simulink library "Lib_CanCommunication"  (R2019b)
settings: Solver=VariableStepAuto  StartTime=0.0  StopTime=10.0  RelTol=1e-3
PostLoadFcn:
  | , if any(exist('dsrtsu_mdlpostloadfcn', 'file') == [2, 3, 6]), try dsrtsu_mdlpostloadfcn('Execute', bdroot); catch fprintf('Error in PostLoadFcn (dsrtsu_mdlpostloadfcn) for model "%s":\n %s\n', bdroot, lasterr); end, end,
undefined symbols (not defined in the file): Counter, CRC, default_customer_can_bus, default_vehicle_state_bus, LateralAcceleration, LongitudinalAcceleration, Motion, Powertrain_1, Steering, steering_angle_range_rad_to_steering_wheel_angle_range_deg_gain, SteeringWheelAngle, SteeringWheelAngleSign, SteeringWheelSpeed, SteeringWheelSpeedSign, SteeringWheelTorque, SteeringWheelTorqueSign, VehicleVelocity, YawRate, YawRateSign
libraries: rtican x8, simulink x6
(part 2 of 3)

== system Lib_CanCommunication/CanCommunication/VehicleCAN/Powertrain_1Message ==
  Bus Creator : BusCreator  Inputs=8  OutDataTypeStr=Bus: Powertrain_1  NonVirtualBus=on
  Powertrain_1 : rtican/RTICAN Receive (RX)   Reserved1=[]  Reserved2=[]  Reserved3=[]  Reserved4=[]  SfcnMessage=[]  Msg_Struct=[]  BoardTypeNo=[]  BoardNo=[]  ChannelNo=[]  Parameters=[]  DialogFcn=[]  UnitName=[]  Revision=[]  UnitValues=[]  DSProperties=struct('RTI',struct('Version',uint32(5),'BlockType',struct('isSLSource',uint8(1),'isSLSink',uint8(1),'isHWSource',uint8(0),'isHWSink',uint8(0),'isSetup',uint8(0),'isInline',uint8(1),'isNonInline',uint8(0),'isInterrupt',uint8(0),'isChannelwise',uint8(0)),'IOBoardType','RTICAN','UnitType','MESSAGE','Identifier','RX','DialogType','MSVC','BlockSet','RTICAN','SlaveProcessor','CAN'))  RTIBlockInterface=struct('OutputPortsWidth',int32([1 1 1 1 1 1 1 1 1 1 1]),'OutputPortsActive',ones(1,11),'OutputPortsName',{{'CRC','Counter','Gear','ThrottlePedalPos','EngineSpeed','ActualTorqueEngine','EngineRunning','RequestedTorqueEngine',['RX status'],['RX time'],['RX delta time']}},'OutputPortsDataType',{{'SS_UINT8','SS_UINT8','SS_UINT8','SS_DOUBLE','SS_DOUBLE','SS_UINT16','SS_BOOLEAN','SS_INT16','SS_DOUBLE','SS_DOUBLE','SS_DOUBLE'}},'OutputPortsLabel',{{'CRC','Counter','Gear','ThrottlePedalPos','EngineSpeed','ActualTorqueEngine','EngineRunning','RequestedTorqueEngine','','',''}},'OutputPortsLabelMode','ON','InputPortsWidth',int32(0),'InputPortsActive',0,'DialogFcn','rtican_message_interface_gui','BlockDisplay',{{'','center'}},'IconTransparency','on','ParameterTunableNames',{{}},'InitLevel',3,'BlockName',struct('Token',{{'Powertrain_1'}}),'SampleTime',{{-1}},'TriggerPort',{{'none'}},'EnablePort',{{'none'}})  RTIBlockParameters="struct('BoardTypeNo',{{1,'OFF',[]}},'BoardNo',{{1,'ON',[1 16]}},'ChannelNo',{{2,'ON',[1 2]}},'Parameters',{{struct('DataFileSupport',struct('DataFileSelectedMaster',1,'DataFileSelectedLocal',0,'DataFileName','c:\\users\\kessler\\documents\\fav\\apollo_opensource\\modules\\dbc\\vehicledata_can_tfd7-17008-03_fortiss_gte.dbc|','DataFileDate',{{{''}}},'SelectedFile',['<no file selected>']),'Options',struct('StatusSelected',1,'TimeSelected',1,'DeltaTimeSelected',1,'BytePortSelected',0,'MessageLengthSelected',0,'TriggerPort',struct('Selected',0,'TriggerType',0),'UserCoding',struct('Selected',0,'InterfaceFile','UserDecodingFile','FcnName','UserDecodeFcn','InportSelected',0,'InportWidth',1,'OutportSelected',0,'OutportWidth',1),'EnablePortSelected',0,'SignalOnPortnameSelected',1,'UseRXService',0),'Message',struct('MsgOnBlocknameSelected',1,'MsgName','Powertrain_1','MsgIdFormat',0,'MsgId',4,'MsgLength',8,'NumSignals',8,'SampleTime',-1,'Signal',struct('SgnName',{'CRC','Counter','Gear','ThrottlePedalPos','EngineSpeed','ActualTorqueEngine','EngineRunning','RequestedTorqueEngine'},'SgnStartBit',{0,8,12,16,24,40,51,52},'SgnLength',{8,4,4,8,16,11,1,12},'SgnType',{0,0,0,0,0,0,0,0},'ModeValue',{-1,-1,-1,-1,-1,-1,-1,-1},'DataType',{0,0,0,0,0,0,0,0},'ByteLayout',{0,0,0,0,0,0,0,0},'Factor',{1,1,1,0.4,2^-2,1,1,1},'Offset',{0,0,0,0,0,0,0,-1527},'SgnComment',{{['Checksum for Powertrain_1 message:  CRC = Byte1 XOR Byte2 XOR Byte3 XOR Byte4 XOR Byte5 XOR Byte6 XOR Byte7. ']},{['Counter for Powertrain_1 message, incremented with every transmittal and periodically running from 0 to 15.']},{['Currently engaged gear. ']},{['Relative position of the throttle pedal in percent (100% = kickdown). ']},{['Engine speed in rpm. ']},{['Engine torque in Nm which is displayed in instrument cluster.']},{['Engine state.']},{['Engine torque requested by driver or ACC.']}},'SgnUnit',{'-','-','-','%','rpm','Nm','-','Nm'},'Min',{0,0,0,0,0,0,0,-1527},'Max',{255,15,15,101.6,16383,2045,1,1527},'SLDataType',{'SS_UINT8','SS_UINT8','SS_UINT8','SS_DOUBLE','SS_DOUBLE','SS_UINT16','SS_BOOLEAN','SS_INT16'}),'MsgIdNumFormat',0,'MsgComment',{{['Engine-related information.']}}),'Version',1.2,'general',struct('isFromLib',0)),'OFF',[]}},'GroupId',{{struct('Group',{{'RTICAN'}},'No',1,'Behavior',{{'NAMECHANGE'}},'BlockType',{{'SINK'}},'NameChangeFlag',0),'OFF',[]}},'SFcnRTICANMessage',{{struct('MsgType','RX','SFcnPortType','Scalar','MsgName','Powertrain_1','MsgIdFormat','STD','MsgId',4,'MsgLength',8,'NumSignals',8,'SampleTime',-1,'Signal',struct('SgnName',{'CRC','Counter','Gear','ThrottlePedalPos','EngineSpeed','ActualTorqueEngine','EngineRunning','RequestedTorqueEngine'},'SgnStartBit',{0,8,12,16,24,40,51,52},'SgnLength',{8,4,4,8,16,11,1,12},'SgnType',{'standard','standard','standard','standard','standard','standard','standard','standard'},'ModeValue',{-1,-1,-1,-1,-1,-1,-1,-1},'DataType',{['unsigned int'],['unsigned int'],['unsigned int'],['unsigned int'],['unsigned int'],['unsigned int'],['unsigned int'],['unsigned int']},'ByteLayout',{['little endian'],['little endian'],['little endian'],['little endian'],['little endian'],['little endian'],['little endian'],['little endian']},'Factor',{1,1,1,0.4,2^-2,1,1,1},'Offset',{0,0,0,0,0,0,0,-1527},'SLDataType',{'SS_UINT8','SS_UINT8','SS_UINT8','SS_DOUBLE','SS_DOUBLE','SS_UINT16','SS_BOOLEAN','SS_INT16'}),'StatusSelected','yes','TimeSelected','yes','DeltaTimeSelected','yes','BytePortSelected','no','MessageLengthSelected','no','TriggerPort',struct('Selected','no','TriggerType',0),'UserCoding',struct('Selected','no','InterfaceFile','UserDecodingFile','FcnName','UserDecodeFcn','InportSelected','no','InportWidth',1,'OutportSelected','no','OutportWidth',1),'EnablePortSelected','no','UseRXService','no','BoardType','DS1','BoardNo',1,'ControllerNo',2),'OFF',[]}},'TLCFileName',{{'rtican_rx_message','OFF',[]}})"  RTISFcnParameters=struct('SFcnRTICANMessage','struct','TLCFileName','char')  RTIBlockParaDefault=struct('BoardTypeNo',4302,'BoardNo',1,'ChannelNo',1,'Parameters',struct('DataFileSupport',struct('DataFileSelectedMaster',0,'DataFileSelectedLocal',0,'DataFileName','','DataFileDate','','SelectedFile',['<no file selected>']),'Options',struct('StatusSelected',1,'TimeSelected',1,'DeltaTimeSelected',1,'BytePortSelected',0,'MessageLengthSelected',0,'TriggerPort',struct('Selected',0,'TriggerType','rising'),'UserCoding',struct('Selected',0,'InterfaceFile','UserDecodingFile','FcnName','UserDecodeFcn','InportSelected',0,'InportWidth',1,'OutportSelected',0,'OutportWidth',1),'EnablePortSelected',0,'SignalOnPortnameSelected',1,'UseRXService',0),'Message',struct('MsgOnBlocknameSelected',0,'MsgName',['RX Message'],'MsgIdFormat',0,'MsgId',100,'MsgLength',8,'NumSignals',1,'SampleTime',-1,'Signal',struct('SgnName',['RX signal'],'SgnStartBit',0,'SgnLength',8,'SgnType',0,'ModeValue',-1,'DataType',0,'SLDataType','SS_DOUBLE','ByteLayout',0,'Factor',1,'Offset',0,'Min',0,'Max',255,'SgnComment',{{}},'SgnUnit',''),'MsgIdNumFormat',0,'MsgComment',{{''}}),'Version',1.2,'general',struct('isFromLib',1)),'GroupId',struct('Group',{{'RTICAN'}},'No',1,'Behavior',{{'NAMECHANGE'}},'BlockType',{{'SINK'}},'NameChangeFlag',0),'SFcnRTICANMessage',struct('MsgType','RX','MsgName',['RX Message'],'MsgIdFormat','STD','MsgId',100,'MsgLength',8,'NumSignals',1,'SampleTime',-1,'Signal',struct('SgnName',['RX signal'],'SgnStartBit',0,'SgnLength',8,'SgnType','standard','ModeValue',-1,'DataType',['unsigned int'],'ByteLayout',['little endian'],'SLDataType','SS_DOUBLE','Factor',1,'Offset',0),'StatusSelected','yes','TimeSelected','yes','DeltaTimeSelected','yes','BytePortSelected','no','MessageLengthSelected','no','EnablePortSelected','no','UserCoding',struct('Selected','no','InterfaceFile','UserDecodingFile','FcnName','UserDecodeFcn','InportSelected','no','InportWidth',1,'OutportSelected','no','OutportWidth',1),'TriggerPort',struct('Selected','no','TriggerType','rising'),'UseRXService','no','BoardType','DS4302','BoardNo',1,'ControllerNo',1,'SFcnPortType','Scalar'),'TLCFileName','rtican_rx_message')
      settings: AttributesFormatString=Group Id: RTICAN1\n  SourceProductName=dSPACE RTI CAN Blockset
  Powertrain_1Message : Outport  VectorParamsAs1DForOutWhenUnconnected=off
  status : Outport  Port=2  VectorParamsAs1DForOutWhenUnconnected=off
  t : Outport  Port=3  VectorParamsAs1DForOutWhenUnconnected=off
  deltat : Outport  Port=4  VectorParamsAs1DForOutWhenUnconnected=off
  wires:
  Powertrain_1/4 -> Bus Creator/8  "ThrottlePedalPos"
  Powertrain_1/8 -> Bus Creator/7  "RequestedTorqueEngine"
  Powertrain_1/3 -> Bus Creator/6  "Gear"
  Powertrain_1/5 -> Bus Creator/5  "EngineSpeed"
  Powertrain_1/7 -> Bus Creator/4  "EngineRunning"
  Powertrain_1/2 -> Bus Creator/3  "Counter"
  Powertrain_1/1 -> Bus Creator/2  "CRC"
  Powertrain_1/6 -> Bus Creator/1  "ActualTorqueEngine"
  Bus Creator/1 -> Powertrain_1Message/1  "Motion"
  Powertrain_1/10 -> t/1
  Powertrain_1/9 -> status/1
  Powertrain_1/11 -> deltat/1

== system Lib_CanCommunication/CanCommunication/VehicleCAN/SteeringMessage ==
  Bus Creator : BusCreator  Inputs=CRC,Counter,SteeringWheelAngle,SteeringWheelAngleSign,SteeringWheelSpeed,SteeringWheelSpeedSign,SteeringWheelTorque,SteeringWheelTorqueSign  OutDataTypeStr=Bus: Steering  NonVirtualBus=on
  Steering : rtican/RTICAN Receive (RX)   Reserved1=[]  Reserved2=[]  Reserved3=[]  Reserved4=[]  SfcnMessage=[]  Msg_Struct=[]  BoardTypeNo=[]  BoardNo=[]  ChannelNo=[]  Parameters=[]  DialogFcn=[]  UnitName=[]  Revision=[]  UnitValues=[]  DSProperties=struct('RTI',struct('Version',uint32(5),'BlockType',struct('isSLSource',uint8(1),'isSLSink',uint8(1),'isHWSource',uint8(0),'isHWSink',uint8(0),'isSetup',uint8(0),'isInline',uint8(1),'isNonInline',uint8(0),'isInterrupt',uint8(0),'isChannelwise',uint8(0)),'IOBoardType','RTICAN','UnitType','MESSAGE','Identifier','RX','DialogType','MSVC','BlockSet','RTICAN','SlaveProcessor','CAN'))  RTIBlockInterface=struct('OutputPortsWidth',int32([1 1 1 1 1 1 1 1 1 1 1]),'OutputPortsActive',ones(1,11),'OutputPortsName',{{'CRC','Counter','SteeringWheelAngleSign','SteeringWheelSpeedSign','SteeringWheelTorqueSign','SteeringWheelTorque','SteeringWheelAngle','SteeringWheelSpeed',['RX status'],['RX time'],['RX delta time']}},'OutputPortsDataType',{{'SS_UINT8','SS_UINT8','SS_BOOLEAN','SS_BOOLEAN','SS_BOOLEAN','SS_DOUBLE','SS_DOUBLE','SS_UINT16','SS_DOUBLE','SS_DOUBLE','SS_DOUBLE'}},'OutputPortsLabel',{{'CRC','Counter','SteeringWheelAngleSign','SteeringWheelSpeedSign','SteeringWheelTorqueSign','SteeringWheelTorque','SteeringWheelAngle','SteeringWheelSpeed','','',''}},'OutputPortsLabelMode','ON','InputPortsWidth',int32(0),'InputPortsActive',0,'DialogFcn','rtican_message_interface_gui','BlockDisplay',{{'','center'}},'IconTransparency','on','ParameterTunableNames',{{}},'InitLevel',3,'BlockName',struct('Token',{{'Steering'}}),'SampleTime',{{-1}},'TriggerPort',{{'none'}},'EnablePort',{{'none'}})  RTIBlockParameters="struct('BoardTypeNo',{{1,'OFF',[]}},'BoardNo',{{1,'ON',[1 16]}},'ChannelNo',{{2,'ON',[1 2]}},'Parameters',{{struct('DataFileSupport',struct('DataFileSelectedMaster',1,'DataFileSelectedLocal',1,'DataFileName','c:\\users\\esterle\\documents\\repositories\\stack\\src\\autobox\\simulink\\dbc\\vehicledata_can_tfd7-17008-03_fortiss_gte.dbc|','DataFileDate',{{{['06-Jul-2018 10:05:43']},{['06-Jul-2018 10:06:03']}}},'SelectedFile','..\\dbc\\vehicledata_can_tfd7-17008-03_fortiss_gte.dbc'),'Options',struct('StatusSelected',1,'TimeSelected',1,'DeltaTimeSelected',1,'BytePortSelected',0,'MessageLengthSelected',0,'TriggerPort',struct('Selected',0,'TriggerType',0),'UserCoding',struct('Selected',0,'InterfaceFile','UserDecodingFile','FcnName','UserDecodeFcn','InportSelected',0,'InportWidth',1,'OutportSelected',0,'OutportWidth',1),'EnablePortSelected',0,'SignalOnPortnameSelected',1,'UseRXService',0),'Message',struct('MsgOnBlocknameSelected',1,'MsgName','Steering','MsgIdFormat',0,'MsgId',2,'MsgLength',6,'NumSignals',8,'SampleTime',-1,'Signal',struct('SgnName',{'CRC','Counter','SteeringWheelAngleSign','SteeringWheelSpeedSign','SteeringWheelTorqueSign','SteeringWheelTorque','SteeringWheelAngle','SteeringWheelSpeed'},'SgnStartBit',{0,8,12,13,14,15,25,38},'SgnLength',{8,4,1,1,1,10,13,9},'SgnType',{0,0,0,0,0,0,0,0},'ModeValue',{-1,-1,-1,-1,-1,-1,-1,-1},'DataType',{0,0,0,0,0,0,0,0},'ByteLayout',{0,0,0,0,0,0,0,0},'Factor',{1,1,1,1,1,0.01,0.1,5},'Offset',{0,0,0,0,0,0,0,0},'SgnComment',{{['Checksum for Steering message:  CRC = Byte1 XOR Byte2 XOR Byte3 XOR Byte4 XOR Byte5. ']},{['Counter for Steering message, incremented with every transmittal and periodically running from 0 to 15.']},{['Sign of the absolute position of the steering wheel.']},{['Sign of the steering wheel turning speed.']},{['Sign of the applied steering wheel torque.']},{['Current absolute torque applied to the steering wheel.']},{['Current absolute position of the steering wheel.']},{['Current absolute turning speed of the steering wheel.']}},'SgnUnit',{'-','-','-','-','-','Nm','deg','deg/s'},'Min',{0,0,0,0,0,0,0,0},'Max',{255,15,1,1,1,8,800,2500},'SLDataType',{'SS_UINT8','SS_UINT8','SS_BOOLEAN','SS_BOOLEAN','SS_BOOLEAN','SS_DOUBLE','SS_DOUBLE','SS_UINT16'}),'MsgIdNumFormat',0,'MsgComment',{{['Steering wheel information. ']}}),'Version',1.2,'general',struct('isFromLib',0)),'OFF',[]}},'GroupId',{{struct('Group',{{'RTICAN'}},'No',3,'Behavior',{{'NAMECHANGE'}},'BlockType',{{'SINK'}},'NameChangeFlag',0),'OFF',[]}},'SFcnRTICANMessage',{{struct('MsgType','RX','SFcnPortType','Scalar','MsgName','Steering','MsgIdFormat','STD','MsgId',2,'MsgLength',6,'NumSignals',8,'SampleTime',-1,'Signal',struct('SgnName',{'CRC','Counter','SteeringWheelAngleSign','SteeringWheelSpeedSign','SteeringWheelTorqueSign','SteeringWheelTorque','SteeringWheelAngle','SteeringWheelSpeed'},'SgnStartBit',{0,8,12,13,14,15,25,38},'SgnLength',{8,4,1,1,1,10,13,9},'SgnType',{'standard','standard','standard','standard','standard','standard','standard','standard'},'ModeValue',{-1,-1,-1,-1,-1,-1,-1,-1},'DataType',{['unsigned int'],['unsigned int'],['unsigned int'],['unsigned int'],['unsigned int'],['unsigned int'],['unsigned int'],['unsigned int']},'ByteLayout',{['little endian'],['little endian'],['little endian'],['little endian'],['little endian'],['little endian'],['little endian'],['little endian']},'Factor',{1,1,1,1,1,0.01,0.1,5},'Offset',{0,0,0,0,0,0,0,0},'SLDataType',{'SS_UINT8','SS_UINT8','SS_BOOLEAN','SS_BOOLEAN','SS_BOOLEAN','SS_DOUBLE','SS_DOUBLE','SS_UINT16'}),'StatusSelected','yes','TimeSelected','yes','DeltaTimeSelected','yes','BytePortSelected','no','MessageLengthSelected','no','TriggerPort',struct('Selected','no','TriggerType',0),'UserCoding',struct('Selected','no','InterfaceFile','UserDecodingFile','FcnName','UserDecodeFcn','InportSelected','no','InportWidth',1,'OutportSelected','no','OutportWidth',1),'EnablePortSelected','no','UseRXService','no','BoardType','DS1','BoardNo',1,'ControllerNo',2),'OFF',[]}},'TLCFileName',{{'rtican_rx_message','OFF',[]}})"  RTISFcnParameters=struct('SFcnRTICANMessage','struct','TLCFileName','char')  RTIBlockParaDefault=struct('BoardTypeNo',4302,'BoardNo',1,'ChannelNo',1,'Parameters',struct('DataFileSupport',struct('DataFileSelectedMaster',0,'DataFileSelectedLocal',0,'DataFileName','','DataFileDate','','SelectedFile',['<no file selected>']),'Options',struct('StatusSelected',1,'TimeSelected',1,'DeltaTimeSelected',1,'BytePortSelected',0,'MessageLengthSelected',0,'TriggerPort',struct('Selected',0,'TriggerType','rising'),'UserCoding',struct('Selected',0,'InterfaceFile','UserDecodingFile','FcnName','UserDecodeFcn','InportSelected',0,'InportWidth',1,'OutportSelected',0,'OutportWidth',1),'EnablePortSelected',0,'SignalOnPortnameSelected',1,'UseRXService',0),'Message',struct('MsgOnBlocknameSelected',0,'MsgName',['RX Message'],'MsgIdFormat',0,'MsgId',100,'MsgLength',8,'NumSignals',1,'SampleTime',-1,'Signal',struct('SgnName',['RX signal'],'SgnStartBit',0,'SgnLength',8,'SgnType',0,'ModeValue',-1,'DataType',0,'SLDataType','SS_DOUBLE','ByteLayout',0,'Factor',1,'Offset',0,'Min',0,'Max',255,'SgnComment',{{}},'SgnUnit',''),'MsgIdNumFormat',0,'MsgComment',{{''}}),'Version',1.2,'general',struct('isFromLib',1)),'GroupId',struct('Group',{{'RTICAN'}},'No',1,'Behavior',{{'NAMECHANGE'}},'BlockType',{{'SINK'}},'NameChangeFlag',0),'SFcnRTICANMessage',struct('MsgType','RX','MsgName',['RX Message'],'MsgIdFormat','STD','MsgId',100,'MsgLength',8,'NumSignals',1,'SampleTime',-1,'Signal',struct('SgnName',['RX signal'],'SgnStartBit',0,'SgnLength',8,'SgnType','standard','ModeValue',-1,'DataType',['unsigned int'],'ByteLayout',['little endian'],'SLDataType','SS_DOUBLE','Factor',1,'Offset',0),'StatusSelected','yes','TimeSelected','yes','DeltaTimeSelected','yes','BytePortSelected','no','MessageLengthSelected','no','EnablePortSelected','no','UserCoding',struct('Selected','no','InterfaceFile','UserDecodingFile','FcnName','UserDecodeFcn','InportSelected','no','InportWidth',1,'OutportSelected','no','OutportWidth',1),'TriggerPort',struct('Selected','no','TriggerType','rising'),'UseRXService','no','BoardType','DS4302','BoardNo',1,'ControllerNo',1,'SFcnPortType','Scalar'),'TLCFileName','rtican_rx_message')
      settings: AttributesFormatString=Group Id: RTICAN3\n  SourceProductName=dSPACE RTI CAN Blockset
  SteeringMessage : Outport  VectorParamsAs1DForOutWhenUnconnected=off
  status : Outport  Port=2  VectorParamsAs1DForOutWhenUnconnected=off
  t : Outport  Port=3  VectorParamsAs1DForOutWhenUnconnected=off
  dt : Outport  Port=4  VectorParamsAs1DForOutWhenUnconnected=off
  wires:
  Steering/9 -> status/1
  Steering/10 -> t/1
  Steering/11 -> dt/1
  Bus Creator/1 -> SteeringMessage/1  "Steering"
  Steering/1 -> Bus Creator/1  "CRC"
  Steering/2 -> Bus Creator/2  "Counter"
  Steering/3 -> Bus Creator/4  "SteeringWheelAngleSign"
  Steering/4 -> Bus Creator/6  "SteeringWheelSpeedSign"
  Steering/5 -> Bus Creator/8  "SteeringWheelTorqueSign"
  Steering/6 -> Bus Creator/7  "SteeringWheelTorque"
  Steering/7 -> Bus Creator/3  "SteeringWheelAngle"
  Steering/8 -> Bus Creator/5  "SteeringWheelSpeed"

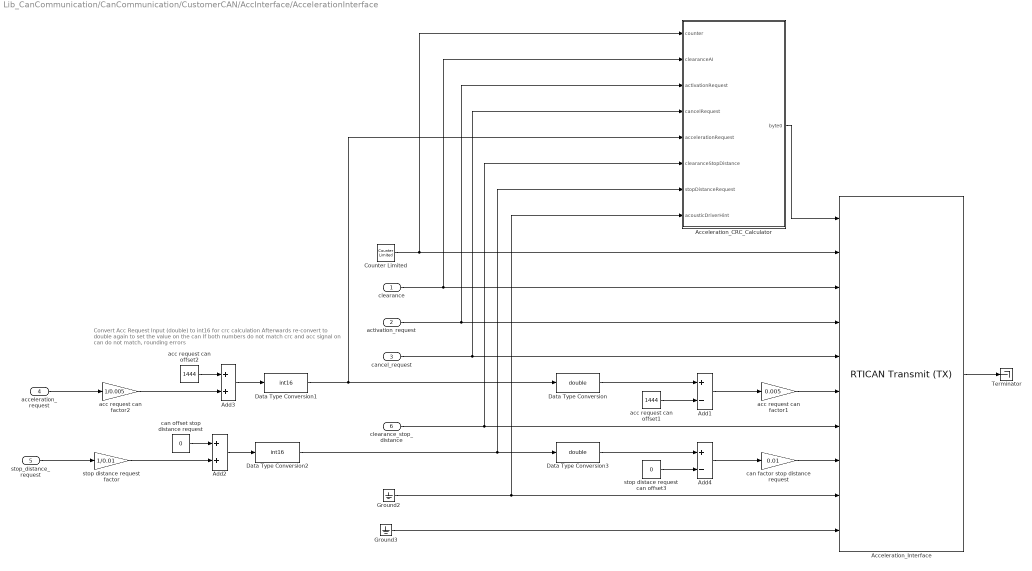
== system Lib_CanCommunication/CanCommunication/CustomerCAN/AccInterface/AccelerationInterface ==
  note: Convert Acc Request Input (double) to int16 for crc calculation
      | Afterwards re-convert to double again to set the value on the can
      | If both numbers do not match crc and acc signal on can do not match, rounding errors
  clearance : Inport
  activation_request : Inport  Port=2
  cancel_request : Inport  Port=3
  acceleration_request : Inport  Port=4
  stop_distance_request : Inport  Port=5
  clearance_stop_distance : Inport  Port=6
  Acceleration_CRC_Calculator : MATLAB Function  TreatAsAtomicUnit=on
  Acceleration_Interface : rtican/RTICAN Transmit (TX)   Reserved1=[]  Reserved2=[]  Reserved3=[]  Reserved4=[]  SfcnMessage=[]  Msg_Struct=[]  BoardTypeNo=[]  BoardNo=[]  ChannelNo=[]  Parameters=[]  DialogFcn=[]  UnitName=[]  Revision=[]  UnitValues=[]  DSProperties=struct('RTI',struct('Version',uint32(5),'BlockType',struct('isSLSource',uint8(1),'isSLSink',uint8(1),'isHWSource',uint8(0),'isHWSink',uint8(0),'isSetup',uint8(0),'isInline',uint8(1),'isNonInline',uint8(0),'isInterrupt',uint8(0),'isChannelwise',uint8(0)),'IOBoardType','RTICAN','UnitType','MESSAGE','Identifier','TX','DialogType','MSVC','BlockSet','RTICAN','SlaveProcessor','CAN'))  RTIBlockInterface=struct('InputPortsWidth',int32([1 1 1 1 1 1 1 1 1 1]),'InputPortsActive',[1 1 1 1 1 1 1 1 1 1],'InputPortsName',{{'CRC','Counter','ClearanceAI','ActivationRequest','CancelRequest','AccelerationRequest','ClearanceStopDistance','StopDistanceRequest','AcousticDriverHint','OpticalDriverHint'}},'InputPortsDataType',{{'SS_UINT8','SS_UINT8','SS_BOOLEAN','SS_BOOLEAN','SS_BOOLEAN','SS_DOUBLE','SS_BOOLEAN','SS_DOUBLE','SS_UINT8','SS_BOOLEAN'}},'OutputPortsWidth',int32(1),'OutputPortsActive',1,'OutputPortsName',{{['TX status']}},'DialogFcn','rtican_message_interface_gui','BlockDisplay',{{'','center'}},'IconTransparency','on','InitLevel',3,'BlockName',struct('Token',{{'Acceleration_Interface'}}),'SampleTime',{{0.02}},'TriggerPort',{{'none'}},'EnablePort',{{'none'}})  RTIBlockParameters=struct('BoardTypeNo',{{1,'OFF',[]}},'BoardNo',{{1,'ON',[1 16]}},'ChannelNo',{{1,'ON',[1 2]}},'Parameters',{{struct('DataFileSupport',struct('DataFileSelectedMaster',1,'DataFileSelectedLocal',1,'DataFileName','c:\fav\stack\src\autobox\simulink\dbc\customer_can_tfd7-17008-03_fortiss_gte.dbc|','DataFileDate',{{{['03-Aug-2018 07:53:06']}}},'SelectedFile','..\dbc\customer_can_tfd7-17008-03_fortiss_gte.dbc'),'Options',struct('StatusSelected',1,'TimeSelected',0,'DeltaTimeSelected',0,'DelayTimeSelected',0,'DelayTimeTXCommandSelected',0,'EncodeSetUnusedBitsToOne',0,'EnableMsgLoopback',0,'TriggerPort',struct('Selected',0,'TriggerType',0),'EnablePortSelected',0,'SignalOnPortnameSelected',1,'UserCoding',struct('Selected',0,'InterfaceFile','UserEncodingFile','FcnName','UserEncodeFcn','InportSelected',0,'InportWidth',1,'OutportSelected',0,'OutportWidth',1),'TerminationMsg',struct('Selected',0,'Byte0_7','0'),'InitialMsg',struct('Selected',0,'Byte0_7','0')),'Message',struct('MsgOnBlocknameSelected',1,'MsgName','Acceleration_Interface','MsgIdFormat',0,'MsgId',256,'MsgLength',6,'NumSignals',10,'SampleTime',0.02,'StartTime',struct('Selected',0,'Value',1),'AutoRepeatTime',struct('Selected',0,'Value',0.1),'Timeout',struct('Selected',0,'Value',0.1),'DelayTime',struct('Selected',0,'Value',0.1),'Signal',struct('SgnName',{'CRC','Counter','ClearanceAI','ActivationRequest','CancelRequest','AccelerationRequest','ClearanceStopDistance','StopDistanceRequest','AcousticDriverHint','OpticalDriverHint'},'SgnStartBit',{0,8,12,13,14,15,26,27,38,40},'SgnLength',{8,4,1,1,1,11,1,11,2,1},'SgnType',{0,0,0,0,0,0,0,0,0,0},'ModeValue',{-1,-1,-1,-1,-1,-1,-1,-1,-1,-1},'DataType',{0,0,0,0,0,0,0,0,0,0},'ByteLayout',{0,0,0,0,0,0,0,0,0,0},'Factor',{1,1,1,1,1,0.005,1,0.01,1,1},'Offset',{0,0,0,0,0,-7.22,0,0,0,0},'SgnComment',{{['Checksum for AI message: CRC = Byte1 XOR Byte2 XOR Byte3 XOR Byte 4.']},{['Counter for AI message, incremented with every transmittal and periodically running from 0 to 15.']},{['Clearance signal for AI. Has to be transmitted before interface can be activated. ']},{['Activation signal for AI. Has to be transmitted after interface has been cleared. ']},{['For deactivating AI via CAN. ']},{['Acceleration request value in m/s². ']},{['Clearance signal for StopDistance control in the AI. Has to be transmitted before StopDistance value can be requested.']},{['StopDistance request value in m. ']},{['Acoustic driver warning.']},{['Optical driver warning (for future use).']}},'SgnUnit',{'-','-','-','-','-','m/s²','-','m','-','-'},'Min',{0,0,0,0,0,-7.22,0,0,0,0},'Max',{255,15,1,1,1,3.005,1,20.45,3,1},'SLDataType',{'SS_UINT8','SS_UINT8','SS_BOOLEAN','SS_BOOLEAN','SS_BOOLEAN','SS_DOUBLE','SS_BOOLEAN','SS_DOUBLE','SS_UINT8','SS_BOOLEAN'}),'MsgIdNumFormat',0,'MsgComment',{{['Information about the Acceleration Interface. ']}}),'Version',1.2,'general',struct('isFromLib',0)),'OFF',[]}},'GroupId',{{struct('Group',{{'RTICAN'}},'No',2,'Behavior',{{'NAMECHANGE'}},'BlockType',{{'SINK'}},'NameChangeFlag',0),'OFF',[]}},'SFcnRTICANMessage',{{struct('MsgType','TX','SFcnPortType','Scalar','MsgName','Acceleration_Interface','MsgIdFormat','STD','MsgId',256,'MsgLength',6,'NumSignals',10,'SampleTime',0.02,'StartTime',struct('Selected','no','Value',1),'AutoRepeatTime',struct('Selected','no','Value',0.1),'Timeout',struct('Selected','no','Value',0.1),'Signal',struct('SgnName',{'CRC','Counter','ClearanceAI','ActivationRequest','CancelRequest','AccelerationRequest','ClearanceStopDistance','StopDistanceRequest','AcousticDriverHint','OpticalDriverHint'},'SgnStartBit',{0,8,12,13,14,15,26,27,38,40},'SgnLength',{8,4,1,1,1,11,1,11,2,1},'SgnType',{'standard','standard','standard','standard','standard','standard','standard','standard','standard','standard'},'ModeValue',{-1,-1,-1,-1,-1,-1,-1,-1,-1,-1},'DataType',{['unsigned int'],['unsigned int'],['unsigned int'],['unsigned int'],['unsigned int'],['unsigned int'],['unsigned int'],['unsigned int'],['unsigned int'],['unsigned int']},'ByteLayout',{['little endian'],['little endian'],['little endian'],['little endian'],['little endian'],['little endian'],['little endian'],['little endian'],['little endian'],['little endian']},'Factor',{1,1,1,1,1,0.005,1,0.01,1,1},'Offset',{0,0,0,0,0,-7.22,0,0,0,0},'SLDataType',{'SS_UINT8','SS_UINT8','SS_BOOLEAN','SS_BOOLEAN','SS_BOOLEAN','SS_DOUBLE','SS_BOOLEAN','SS_DOUBLE','SS_UINT8','SS_BOOLEAN'}),'StatusSelected','yes','TimeSelected','no','DeltaTimeSelected','no','DelayTimeSelected','no','DelayTimeTXCommandSelected','no','EncodeSetUnusedBitsToOne','no','EnableMsgLoopback','no','TriggerPort',struct('Selected','no','TriggerType',0),'EnablePortSelected','no','UserCoding',struct('Selected','no','InterfaceFile','UserEncodingFile','FcnName','UserEncodeFcn','InportSelected','no','InportWidth',1,'OutportSelected','no','OutportWidth',1),'TerminationMsg',struct('Selected','no','Byte0','0x00','Byte1','0x00','Byte2','0x00','Byte3','0x00','Byte4','0x00','Byte5','0x00','Byte6','0x00','Byte7','0x00'),'InitialMsg',struct('Selected','no','Byte0','0x00','Byte1','0x00','Byte2','0x00','Byte3','0x00','Byte4','0x00','Byte5','0x00','Byte6','0x00','Byte7','0x00'),'BoardType','DS1','BoardNo',1,'ControllerNo',1),'OFF',[]}},'TLCFileName',{{'rtican_tx_message','OFF',[]}})  RTISFcnParameters=struct('SFcnRTICANMessage','struct','TLCFileName','char')  RTIBlockParaDefault=struct('BoardTypeNo',4302,'BoardNo',1,'ChannelNo',1,'Parameters',struct('DataFileSupport',struct('DataFileSelectedMaster',0,'DataFileSelectedLocal',0,'DataFileName','','DataFileDate','','SelectedFile',['<no file selected>']),'Options',struct('StatusSelected',1,'TimeSelected',1,'DeltaTimeSelected',1,'DelayTimeSelected',1,'DelayTimeTXCommandSelected',0,'EncodeSetUnusedBitsToOne',0,'EnableMsgLoopback',0,'TriggerPort',struct('Selected',0,'TriggerType','rising'),'EnablePortSelected',0,'SignalOnPortnameSelected',1,'UserCoding',struct('Selected',0,'InterfaceFile','UserEncodingFile','FcnName','UserEncodeFcn','InportSelected',0,'InportWidth',1,'OutportSelected',0,'OutportWidth',1),'TerminationMsg',struct('Selected',0,'Byte0_7','0'),'InitialMsg',struct('Selected',0,'Byte0_7','0')),'Message',struct('MsgOnBlocknameSelected',0,'MsgName',['TX Message'],'MsgIdFormat',0,'MsgId',100,'MsgLength',8,'NumSignals',1,'SampleTime',-1,'StartTime',struct('Selected',0,'Value',0),'AutoRepeatTime',struct('Selected',0,'Value',0.1),'Timeout',struct('Selected',0,'Value',0.1),'DelayTime',struct('Selected',0,'Value',0.1),'Signal',struct('SgnName',['TX signal'],'SgnStartBit',0,'SgnLength',8,'SgnType',0,'ModeValue',-1,'DataType',0,'SLDataType','SS_DOUBLE','ByteLayout',0,'Factor',1,'Offset',0,'Min',0,'Max',255,'SgnComment',{{}},'SgnUnit',''),'MsgIdNumFormat',0,'MsgComment',{{''}}),'Version',1.2,'general',struct('isFromLib',1)),'GroupId',struct('Group',{{'RTICAN'}},'No',1,'Behavior',{{'NAMECHANGE'}},'BlockType',{{'SINK'}},'NameChangeFlag',0),'SFcnRTICANMessage',struct('MsgType','TX','MsgName',['TX Message'],'MsgIdFormat','STD','MsgId',100,'MsgLength',2,'NumSignals',1,'SampleTime',-1,'StartTime',struct('Selected','no','Value',0),'AutoRepeatTime',struct('Selected','no','Value',0.1),'Timeout',struct('Selected','no','Value',0.1),'DelayTime',struct('Selected','no','Value',0.1),'Signal',struct('SgnName',['TX signal'],'SgnStartBit',0,'SgnLength',8,'SgnType','standard','ModeValue',-1,'DataType',['unsigned int'],'ByteLayout',['little endian'],'SLDataType','SS_DOUBLE','Factor',1,'Offset',0),'StatusSelected','yes','TimeSelected','yes','DeltaTimeSelected','yes','DelayTimeSelected','yes','EnablePortSelected','no','EnableMsgLoopback','no','DelayTimeTXCommandSelected','no','EncodeSetUnusedBitsToOne','no','UserCoding',struct('Selected','no','InterfaceFile','UserDecodingFile','FcnName','UserDecodeFcn','InportSelected','no','InportWidth',1,'OutportSelected','no','OutportWidth',1),'TerminationMsg',struct('Selected','no','Byte0','0x00','Byte1','0x00','Byte2','0x00','Byte3','0x00','Byte4','0x00','Byte5','0x00','Byte6','0x00','Byte7','0x00'),'InitialMsg',struct('Selected','no','Byte0','0x00','Byte1','0x00','Byte2','0x00','Byte3','0x00','Byte4','0x00','Byte5','0x00','Byte6','0x00','Byte7','0x00'),'TriggerPort',struct('Selected','no','TriggerType','rising'),'BoardType','DS4302','BoardNo',1,'ControllerNo',1,'SFcnPortType','Scalar'),'TLCFileName','rtican_tx_message')
      settings: AttributesFormatString=Group Id: RTICAN2\n  SourceProductName=dSPACE RTI CAN Blockset
  Add1 : Sum  Inputs=+-
  Add2 : Sum
  Add3 : Sum
  Add4 : Sum  Inputs=+-
  Counter Limited : simulink/Sources/Counter Limited  uplimit=15  tsamp=-1
  Data Type Conversion : DataTypeConversion  OutDataTypeStr=double
  Data Type Conversion1 : DataTypeConversion  OutDataTypeStr=int16
  Data Type Conversion2 : DataTypeConversion  OutDataTypeStr=int16
  Data Type Conversion3 : DataTypeConversion  OutDataTypeStr=double
  Ground2 : Ground
  Ground3 : Ground
  Terminator : Terminator
  acc request can factor1 : Gain  Gain=0.005
  acc request can factor2 : Gain  Gain=1/0.005
  acc request can offset1 : Constant  Value=1444  OutDataTypeStr=Inherit: Inherit via back propagation
  acc request can offset2 : Constant  Value=1444
  can factor stop distance request : Gain  Gain=0.01
  can offset stop distance request : Constant  Value=0
  stop distace request can offset3 : Constant  Value=0  OutDataTypeStr=Inherit: Inherit via back propagation
  stop distance request factor : Gain  Gain=1/0.01
  wires:
  can factor stop distance request/1 -> Acceleration_Interface/8
  Add4/1 -> can factor stop distance request/1
  stop distace request can offset3/1 -> Add4/2
  Data Type Conversion3/1 -> Add4/1
  stop_distance_request/1 -> stop distance request factor/1
  can offset stop distance request/1 -> Add2/1
  Add2/1 -> Data Type Conversion2/1
  stop distance request factor/1 -> Add2/2
  Data Type Conversion/1 -> Add1/1
  Add3/1 -> Data Type Conversion1/1
  acc request can offset2/1 -> Add3/1
  acc request can factor2/1 -> Add3/2
  Add1/1 -> acc request can factor1/1
  acc request can factor1/1 -> Acceleration_Interface/6
  acc request can offset1/1 -> Add1/2
  Data Type Conversion1/1 -> Data Type Conversion/1, Acceleration_CRC_Calculator/5(accelerationRequest)
  acceleration_request/1 -> acc request can factor2/1
  Data Type Conversion2/1 -> Data Type Conversion3/1, Acceleration_CRC_Calculator/7(stopDistanceRequest)
  Acceleration_Interface/1 -> Terminator/1
  clearance_stop_distance/1 -> Acceleration_CRC_Calculator/6(clearanceStopDistance), Acceleration_Interface/7
  activation_request/1 -> Acceleration_Interface/4, Acceleration_CRC_Calculator/3(activationRequest)
  cancel_request/1 -> Acceleration_Interface/5, Acceleration_CRC_Calculator/4(cancelRequest)
  Ground3/1 -> Acceleration_Interface/10
  Ground2/1 -> Acceleration_CRC_Calculator/8(acousticDriverHint), Acceleration_Interface/9
  Acceleration_CRC_Calculator/1(byte0) -> Acceleration_Interface/1
  Counter Limited/1 -> Acceleration_Interface/2, Acceleration_CRC_Calculator/1(counter)
  clearance/1 -> Acceleration_CRC_Calculator/2(clearanceAI), Acceleration_Interface/3

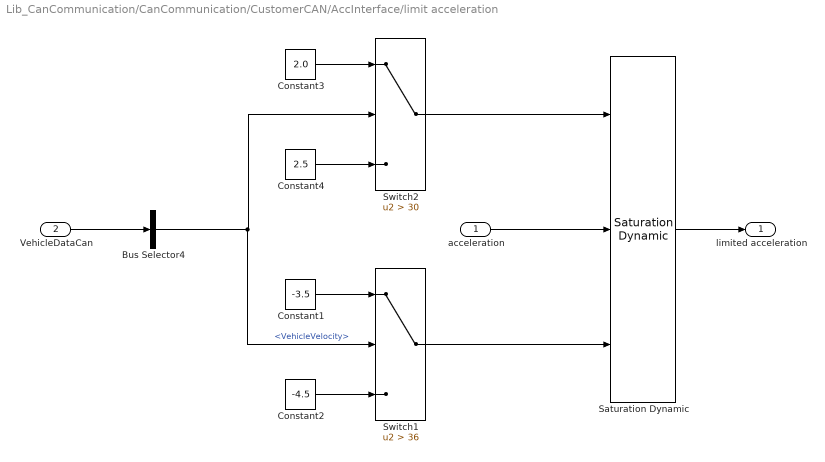
== system Lib_CanCommunication/CanCommunication/CustomerCAN/AccInterface/limit acceleration ==
  acceleration : Inport
  VehicleDataCan : Inport  Port=2
  Bus Selector4 : BusSelector  OutputSignals=Motion.VehicleVelocity
  Constant1 : Constant  Value=-3.5
  Constant2 : Constant  Value=-4.5
  Constant3 : Constant  Value=2.0
  Constant4 : Constant  Value=2.5
  Saturation Dynamic : simulink/Discontinuities/Saturation Dynamic  OutMin=[]  OutMax=[]  OutDataTypeStr=Inherit: Same as second input  OutDataType=fixdt(1, 16)  OutScaling=2^-10  DoSatur=off
  Switch1 : Switch  Criteria=u2 > Threshold  Threshold=36
  Switch2 : Switch  Criteria=u2 > Threshold  Threshold=30
  limited acceleration : Outport  VectorParamsAs1DForOutWhenUnconnected=off
  wires:
  Switch2/1 -> Saturation Dynamic/1
  Constant3/1 -> Switch2/1
  Constant4/1 -> Switch2/3
  acceleration/1 -> Saturation Dynamic/2
  VehicleDataCan/1 -> Bus Selector4/1
  Saturation Dynamic/1 -> limited acceleration/1
  Constant2/1 -> Switch1/3
  Bus Selector4/1 -> Switch2/2, Switch1/2  "<VehicleVelocity>"
  Constant1/1 -> Switch1/1
  Switch1/1 -> Saturation Dynamic/3

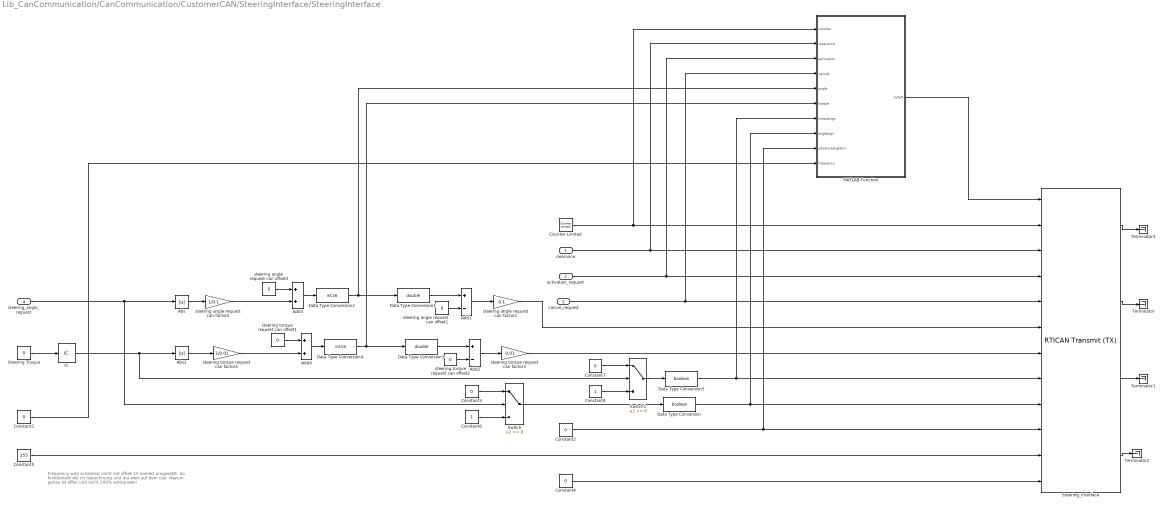
== system Lib_CanCommunication/CanCommunication/CustomerCAN/SteeringInterface/SteeringInterface ==
  note: Frequency wird scheinbar nicht mit offset 15 korrekt umgesetzt.
      | So funktioniert die crc berechnung und der wert auf dem can.
      | Warum genau ist offen und nicht 100% verstanden!
  clearance : Inport
  activation_request : Inport  Port=2
  cancel_request : Inport  Port=3
  steering_angle_request : Inport  Port=4
  Abs : Abs
  Abs2 : Abs
  Add1 : Sum  Inputs=+-
  Add2 : Sum  Inputs=+-
  Add3 : Sum
  Add4 : Sum
  Constant1 : Constant  Value=0  OutMin=0  OutMax=0  OutDataTypeStr=uint8
  Constant2 : Constant  Value=0  OutDataTypeStr=Inherit: Inherit via back propagation
  Constant3 : Constant  Value=0  OutDataTypeStr=boolean
  Constant4 : Constant  Value=0  OutDataTypeStr=Inherit: Inherit via back propagation
  Constant5 : Constant  Value=255  OutDataTypeStr=uint8
  Constant6 : Constant  OutDataTypeStr=boolean
  Constant7 : Constant  Value=0  OutDataTypeStr=boolean
  Constant8 : Constant  OutDataTypeStr=boolean
  Counter Limited : simulink/Sources/Counter Limited  uplimit=15  tsamp=-1
  Data Type Conversion : DataTypeConversion  OutDataTypeStr=boolean
  Data Type Conversion1 : DataTypeConversion  OutDataTypeStr=double
  Data Type Conversion2 : DataTypeConversion  OutDataTypeStr=int16
  Data Type Conversion3 : DataTypeConversion  OutDataTypeStr=double
  Data Type Conversion4 : DataTypeConversion  OutDataTypeStr=int16
  Data Type Conversion5 : DataTypeConversion  OutDataTypeStr=boolean
  IC : InitialCondition  Value=0
  MATLAB Function : MATLAB Function  TreatAsAtomicUnit=on
  Steering Troque : Constant  Value=0  OutDataTypeStr=double
  Steering_Interface : rtican/RTICAN Transmit (TX)   Reserved1=[]  Reserved2=[]  Reserved3=[]  Reserved4=[]  SfcnMessage=[]  Msg_Struct=[]  BoardTypeNo=[]  BoardNo=[]  ChannelNo=[]  Parameters=[]  DialogFcn=[]  UnitName=[]  Revision=[]  UnitValues=[]  DSProperties=struct('RTI',struct('Version',uint32(5),'BlockType',struct('isSLSource',uint8(1),'isSLSink',uint8(1),'isHWSource',uint8(0),'isHWSink',uint8(0),'isSetup',uint8(0),'isInline',uint8(1),'isNonInline',uint8(0),'isInterrupt',uint8(0),'isChannelwise',uint8(0)),'IOBoardType','RTICAN','UnitType','MESSAGE','Identifier','TX','DialogType','MSVC','BlockSet','RTICAN','SlaveProcessor','CAN'))  RTIBlockInterface=struct('InputPortsWidth',int32([1 1 1 1 1 1 1 1 1 1 1 1]),'InputPortsActive',ones(1,12),'InputPortsName',{{'CRC','Counter','ClearanceSI','ActivationRequest','CancelRequest','SteeringAngleRequest','SteeringTorqueRequest','SteeringTorqueRequestSign','SteeringAngleRequestSign','AdvancedSteeringAngleLimitation','Frequency','Amplitude'}},'InputPortsDataType',{{'SS_UINT8','SS_UINT8','SS_UINT8','SS_BOOLEAN','SS_BOOLEAN','SS_DOUBLE','SS_DOUBLE','SS_BOOLEAN','SS_BOOLEAN','SS_BOOLEAN','SS_UINT8','SS_DOUBLE'}},'OutputPortsWidth',int32([1 1 1 1]),'OutputPortsActive',[1 1 1 1],'OutputPortsName',{{['TX status'],['TX time'],['TX delta time'],['TX delay time']}},'DialogFcn','rtican_message_interface_gui','BlockDisplay',{{'','center'}},'IconTransparency','on','InitLevel',3,'BlockName',struct('Token',{{'Steering_Interface'}}),'SampleTime',{{0.02}},'TriggerPort',{{'none'}},'EnablePort',{{'none'}})  RTIBlockParameters=struct('BoardTypeNo',{{1,'OFF',[]}},'BoardNo',{{1,'ON',[1 16]}},'ChannelNo',{{1,'ON',[1 2]}},'Parameters',{{struct('DataFileSupport',struct('DataFileSelectedMaster',1,'DataFileSelectedLocal',1,'DataFileName','c:\fav\stack\src\autobox\simulink\dbc\customer_can_tfd7-17008-03_fortiss_gte.dbc|','DataFileDate',{{{['03-Aug-2018 07:53:06']}}},'SelectedFile','..\dbc\customer_can_tfd7-17008-03_fortiss_gte.dbc'),'Options',struct('StatusSelected',1,'TimeSelected',1,'DeltaTimeSelected',1,'DelayTimeSelected',1,'DelayTimeTXCommandSelected',0,'EncodeSetUnusedBitsToOne',0,'EnableMsgLoopback',0,'TriggerPort',struct('Selected',0,'TriggerType',0),'EnablePortSelected',0,'SignalOnPortnameSelected',1,'UserCoding',struct('Selected',0,'InterfaceFile','UserEncodingFile','FcnName','UserEncodeFcn','InportSelected',0,'InportWidth',1,'OutportSelected',0,'OutportWidth',1),'TerminationMsg',struct('Selected',0,'Byte0_7','0'),'InitialMsg',struct('Selected',0,'Byte0_7','0')),'Message',struct('MsgOnBlocknameSelected',1,'MsgName','Steering_Interface','MsgIdFormat',0,'MsgId',272,'MsgLength',7,'NumSignals',12,'SampleTime',0.02,'StartTime',struct('Selected',0,'Value',7),'AutoRepeatTime',struct('Selected',0,'Value',0.1),'Timeout',struct('Selected',0,'Value',0.1),'DelayTime',struct('Selected',0,'Value',0.1),'Signal',struct('SgnName',{'CRC','Counter','ClearanceSI','ActivationRequest','CancelRequest','SteeringAngleRequest','SteeringTorqueRequest','SteeringTorqueRequestSign','SteeringAngleRequestSign','AdvancedSteeringAngleLimitation','Frequency','Amplitude'},'SgnStartBit',{0,8,12,14,15,16,32,41,42,43,44,48},'SgnLength',{8,4,2,1,1,16,9,1,1,1,4,4},'SgnType',{0,0,0,0,0,0,0,0,0,0,0,0},'ModeValue',{-1,-1,-1,-1,-1,-1,-1,-1,-1,-1,-1,-1},'DataType',{0,0,0,0,0,0,0,0,0,0,0,0},'ByteLayout',{0,0,0,0,0,0,0,0,0,0,0,0},'Factor',{1,1,1,1,1,0.1,0.01,1,1,1,1,2^-1},'Offset',{0,0,0,0,0,0,0,0,0,0,15,0},'SgnComment',{{['Checksum for SI message CRC = Byte1 XOR Byte2 XOR Byte3 XOR Byte4 XOR Byte5.']},{['Counter for SI message, incremented with every transmittal and periodically running from 0 to 15.']},{['Clearance signal for SI. Has to be transmitted before interface can be activated. ']},{['Activation signal for SI. Has to be transmitted after interface has been cleared. ']},{['For deactivating SI via CAN. ']},{['Steering angle request in °.']},{['Steering torque request in Nm. ']},{['Sign of the steering torque request.']},{['Sign of the steering angle request.']},{['Clearance signal for activation of advanced steering angle limitation (for future use).']},{['Frequency of the steering wheel vibration (for future use).']},{['Amplitude of the steering wheel vibration (for future use).']}},'SgnUnit',{'-','-','-','-','-','deg','Nm','-','-','-','Hz','Nm'},'Min',{0,0,0,0,0,0,0,0,0,0,15,0},'Max',{255,15,3,1,1,6553.5,5.11,1,1,1,30,7.5},'SLDataType',{'SS_UINT8','SS_UINT8','SS_UINT8','SS_BOOLEAN','SS_BOOLEAN','SS_DOUBLE','SS_DOUBLE','SS_BOOLEAN','SS_BOOLEAN','SS_BOOLEAN','SS_UINT8','SS_DOUBLE'}),'MsgIdNumFormat',0,'MsgComment',{{['Information about the Steering Interface. ']}}),'Version',1.2,'general',struct('isFromLib',0)),'OFF',[]}},'GroupId',{{struct('Group',{{'RTICAN'}},'No',2,'Behavior',{{'NAMECHANGE'}},'BlockType',{{'SINK'}},'NameChangeFlag',0),'OFF',[]}},'SFcnRTICANMessage',{{struct('MsgType','TX','SFcnPortType','Scalar','MsgName','Steering_Interface','MsgIdFormat','STD','MsgId',272,'MsgLength',7,'NumSignals',12,'SampleTime',0.02,'StartTime',struct('Selected','no','Value',7),'AutoRepeatTime',struct('Selected','no','Value',0.1),'Timeout',struct('Selected','no','Value',0.1),'Signal',struct('SgnName',{'CRC','Counter','ClearanceSI','ActivationRequest','CancelRequest','SteeringAngleRequest','SteeringTorqueRequest','SteeringTorqueRequestSign','SteeringAngleRequestSign','AdvancedSteeringAngleLimitation','Frequency','Amplitude'},'SgnStartBit',{0,8,12,14,15,16,32,41,42,43,44,48},'SgnLength',{8,4,2,1,1,16,9,1,1,1,4,4},'SgnType',{'standard','standard','standard','standard','standard','standard','standard','standard','standard','standard','standard','standard'},'ModeValue',{-1,-1,-1,-1,-1,-1,-1,-1,-1,-1,-1,-1},'DataType',{['unsigned int'],['unsigned int'],['unsigned int'],['unsigned int'],['unsigned int'],['unsigned int'],['unsigned int'],['unsigned int'],['unsigned int'],['unsigned int'],['unsigned int'],['unsigned int']},'ByteLayout',{['little endian'],['little endian'],['little endian'],['little endian'],['little endian'],['little endian'],['little endian'],['little endian'],['little endian'],['little endian'],['little endian'],['little endian']},'Factor',{1,1,1,1,1,0.1,0.01,1,1,1,1,2^-1},'Offset',{0,0,0,0,0,0,0,0,0,0,15,0},'SLDataType',{'SS_UINT8','SS_UINT8','SS_UINT8','SS_BOOLEAN','SS_BOOLEAN','SS_DOUBLE','SS_DOUBLE','SS_BOOLEAN','SS_BOOLEAN','SS_BOOLEAN','SS_UINT8','SS_DOUBLE'}),'StatusSelected','yes','TimeSelected','yes','DeltaTimeSelected','yes','DelayTimeSelected','yes','DelayTimeTXCommandSelected','no','EncodeSetUnusedBitsToOne','no','EnableMsgLoopback','no','TriggerPort',struct('Selected','no','TriggerType',0),'EnablePortSelected','no','UserCoding',struct('Selected','no','InterfaceFile','UserEncodingFile','FcnName','UserEncodeFcn','InportSelected','no','InportWidth',1,'OutportSelected','no','OutportWidth',1),'TerminationMsg',struct('Selected','no','Byte0','0x00','Byte1','0x00','Byte2','0x00','Byte3','0x00','Byte4','0x00','Byte5','0x00','Byte6','0x00','Byte7','0x00'),'InitialMsg',struct('Selected','no','Byte0','0x00','Byte1','0x00','Byte2','0x00','Byte3','0x00','Byte4','0x00','Byte5','0x00','Byte6','0x00','Byte7','0x00'),'BoardType','DS1','BoardNo',1,'ControllerNo',1),'OFF',[]}},'TLCFileName',{{'rtican_tx_message','OFF',[]}})  RTISFcnParameters=struct('SFcnRTICANMessage','struct','TLCFileName','char')  RTIBlockParaDefault=struct('BoardTypeNo',4302,'BoardNo',1,'ChannelNo',1,'Parameters',struct('DataFileSupport',struct('DataFileSelectedMaster',0,'DataFileSelectedLocal',0,'DataFileName','','DataFileDate','','SelectedFile',['<no file selected>']),'Options',struct('StatusSelected',1,'TimeSelected',1,'DeltaTimeSelected',1,'DelayTimeSelected',1,'DelayTimeTXCommandSelected',0,'EncodeSetUnusedBitsToOne',0,'EnableMsgLoopback',0,'TriggerPort',struct('Selected',0,'TriggerType','rising'),'EnablePortSelected',0,'SignalOnPortnameSelected',1,'UserCoding',struct('Selected',0,'InterfaceFile','UserEncodingFile','FcnName','UserEncodeFcn','InportSelected',0,'InportWidth',1,'OutportSelected',0,'OutportWidth',1),'TerminationMsg',struct('Selected',0,'Byte0_7','0'),'InitialMsg',struct('Selected',0,'Byte0_7','0')),'Message',struct('MsgOnBlocknameSelected',0,'MsgName',['TX Message'],'MsgIdFormat',0,'MsgId',100,'MsgLength',8,'NumSignals',1,'SampleTime',-1,'StartTime',struct('Selected',0,'Value',0),'AutoRepeatTime',struct('Selected',0,'Value',0.1),'Timeout',struct('Selected',0,'Value',0.1),'DelayTime',struct('Selected',0,'Value',0.1),'Signal',struct('SgnName',['TX signal'],'SgnStartBit',0,'SgnLength',8,'SgnType',0,'ModeValue',-1,'DataType',0,'SLDataType','SS_DOUBLE','ByteLayout',0,'Factor',1,'Offset',0,'Min',0,'Max',255,'SgnComment',{{}},'SgnUnit',''),'MsgIdNumFormat',0,'MsgComment',{{''}}),'Version',1.2,'general',struct('isFromLib',1)),'GroupId',struct('Group',{{'RTICAN'}},'No',1,'Behavior',{{'NAMECHANGE'}},'BlockType',{{'SINK'}},'NameChangeFlag',0),'SFcnRTICANMessage',struct('MsgType','TX','MsgName',['TX Message'],'MsgIdFormat','STD','MsgId',100,'MsgLength',2,'NumSignals',1,'SampleTime',-1,'StartTime',struct('Selected','no','Value',0),'AutoRepeatTime',struct('Selected','no','Value',0.1),'Timeout',struct('Selected','no','Value',0.1),'DelayTime',struct('Selected','no','Value',0.1),'Signal',struct('SgnName',['TX signal'],'SgnStartBit',0,'SgnLength',8,'SgnType','standard','ModeValue',-1,'DataType',['unsigned int'],'ByteLayout',['little endian'],'SLDataType','SS_DOUBLE','Factor',1,'Offset',0),'StatusSelected','yes','TimeSelected','yes','DeltaTimeSelected','yes','DelayTimeSelected','yes','EnablePortSelected','no','EnableMsgLoopback','no','DelayTimeTXCommandSelected','no','EncodeSetUnusedBitsToOne','no','UserCoding',struct('Selected','no','InterfaceFile','UserDecodingFile','FcnName','UserDecodeFcn','InportSelected','no','InportWidth',1,'OutportSelected','no','OutportWidth',1),'TerminationMsg',struct('Selected','no','Byte0','0x00','Byte1','0x00','Byte2','0x00','Byte3','0x00','Byte4','0x00','Byte5','0x00','Byte6','0x00','Byte7','0x00'),'InitialMsg',struct('Selected','no','Byte0','0x00','Byte1','0x00','Byte2','0x00','Byte3','0x00','Byte4','0x00','Byte5','0x00','Byte6','0x00','Byte7','0x00'),'TriggerPort',struct('Selected','no','TriggerType','rising'),'BoardType','DS4302','BoardNo',1,'ControllerNo',1,'SFcnPortType','Scalar'),'TLCFileName','rtican_tx_message')
      settings: AttributesFormatString=Group Id: RTICAN2\n  SourceProductName=dSPACE RTI CAN Blockset
  Switch : Switch
  Switch1 : Switch
  Terminator{,1..3} (4 alike) : Terminator
  steering angle  request can offset2 : Constant  Value=0
  steering angle request can factor1 : Gain  Gain=0.1
  steering angle request can factor2 : Gain  Gain=1/0.1
  steering angle request can offset1 : Constant  Value=0  OutDataTypeStr=Inherit: Inherit via back propagation
  steering torque  request can offset1 : Constant  Value=0
  steering torque request can factor3 : Gain  Gain=0.01
  steering torque request can factor4 : Gain  Gain=1/0.01
  steering torque request can offset2 : Constant  Value=0  OutDataTypeStr=Inherit: Inherit via back propagation
  wires:
  Constant7/1 -> Switch1/1
  Constant8/1 -> Switch1/3
  Constant6/1 -> Switch/3
  Constant3/1 -> Switch/1
  Constant1/1 -> MATLAB Function/10(frequency)
  Constant5/1 -> Steering_Interface/11
  steering_angle_request/1 -> Abs/1, Switch/2
  IC/1 -> Abs2/1, Switch1/2
  Steering Troque/1 -> IC/1
  Abs2/1 -> steering torque request can factor4/1
  Abs/1 -> steering angle request can factor2/1
  steering torque request can factor3/1 -> Steering_Interface/7
  Switch1/1 -> Data Type Conversion5/1
  Add4/1 -> Data Type Conversion4/1
  steering torque request can factor4/1 -> Add4/2
  Data Type Conversion3/1 -> Add2/1
  steering torque  request can offset1/1 -> Add4/1
  steering torque request can offset2/1 -> Add2/2
  Add2/1 -> steering torque request can factor3/1
  Data Type Conversion4/1 -> Data Type Conversion3/1, MATLAB Function/6(torque)
  Data Type Conversion2/1 -> MATLAB Function/5(angle), Data Type Conversion1/1
  Add1/1 -> steering angle request can factor1/1
  steering angle request can offset1/1 -> Add1/2
  steering angle  request can offset2/1 -> Add3/1
  Data Type Conversion1/1 -> Add1/1
  steering angle request can factor2/1 -> Add3/2
  Add3/1 -> Data Type Conversion2/1
  Steering_Interface/4 -> Terminator2/1
  Steering_Interface/3 -> Terminator1/1
  Steering_Interface/2 -> Terminator/1
  Switch/1 -> Data Type Conversion/1
  steering angle request can factor1/1 -> Steering_Interface/6
  clearance/1 -> Steering_Interface/3, MATLAB Function/2(clearance)
  activation_request/1 -> Steering_Interface/4, MATLAB Function/3(activation)
  cancel_request/1 -> Steering_Interface/5, MATLAB Function/4(cancel)
  Data Type Conversion5/1 -> Steering_Interface/8, MATLAB Function/7(torquesign)
  Constant2/1 -> Steering_Interface/10, MATLAB Function/9(advanceanglelim)
  Constant4/1 -> Steering_Interface/12
  Steering_Interface/1 -> Terminator3/1
  Counter Limited/1 -> Steering_Interface/2, MATLAB Function/1(counter)
  Data Type Conversion/1 -> Steering_Interface/9, MATLAB Function/8(anglesign)
  MATLAB Function/1(byte0) -> Steering_Interface/1

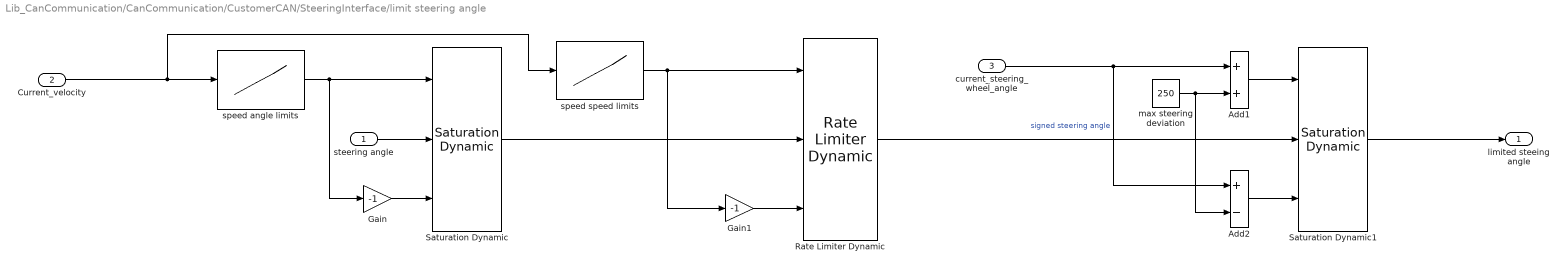
== system Lib_CanCommunication/CanCommunication/CustomerCAN/SteeringInterface/limit steering angle ==
  steering angle : Inport
  Current_velocity : Inport  Port=2
  current_steering_wheel_angle : Inport  Port=3
  Add1 : Sum
  Add2 : Sum  Inputs=+-
  Gain : Gain  Gain=-1
  Gain1 : Gain  Gain=-1
  Rate Limiter Dynamic : simulink/Discontinuities/Rate Limiter Dynamic
      settings: SourceProductName=Simulink
  Saturation Dynamic : simulink/Discontinuities/Saturation Dynamic  OutMin=[]  OutMax=[]  OutDataTypeStr=Inherit: Same as second input  OutDataType=fixdt(1, 16)  OutScaling=2^-10  DoSatur=off
  Saturation Dynamic1 : simulink/Discontinuities/Saturation Dynamic  OutMin=[]  OutMax=[]  OutDataTypeStr=Inherit: Same as second input  OutDataType=fixdt(1, 16)  OutScaling=2^-10  DoSatur=off
  max steering deviation : Constant  Value=250
  speed angle limits : Lookup_n-D  NumberOfTableDimensions=1  BreakpointsForDimension1=[0,10,20,30,40,50,60,70,100,130]  Table=[500,500,350,200,100,60,50,40,30,20]  ExtrapMethod=Clip  UseLastTableValue=on  InternalRulePriority=Speed  RndMeth=Simplest  InputSameDT=on
  speed speed limits : Lookup_n-D  NumberOfTableDimensions=1  BreakpointsForDimension1=[0, 10, 10.01, 200]  Table=[1000, 1000, 260, 260]  ExtrapMethod=Clip  UseLastTableValue=on  InternalRulePriority=Speed  RndMeth=Simplest  InputSameDT=on
  limited steeing angle : Outport  VectorParamsAs1DForOutWhenUnconnected=off
  wires:
  Saturation Dynamic1/1 -> limited steeing angle/1
  max steering deviation/1 -> Add1/2, Add2/2
  Add2/1 -> Saturation Dynamic1/3
  Add1/1 -> Saturation Dynamic1/1
  speed speed limits/1 -> Rate Limiter Dynamic/1, Gain1/1
  Rate Limiter Dynamic/1 -> Saturation Dynamic1/2
  current_steering_wheel_angle/1 -> Add1/1, Add2/1  "signed steering angle"
  Saturation Dynamic/1 -> Rate Limiter Dynamic/2
  Gain/1 -> Saturation Dynamic/3
  speed angle limits/1 -> Saturation Dynamic/1, Gain/1
  steering angle/1 -> Saturation Dynamic/2
  Current_velocity/1 -> speed angle limits/1, speed speed limits/1
  Gain1/1 -> Rate Limiter Dynamic/3
